simulink model "cm_commphasenoise"  (Simulink 10.1)
settings: Solver=FixedStepDiscrete  StartTime=0.0  StopTime=inf  RelTol=1e-3  EnableMultiTasking=on
PreLoadFcn:
  | Nbps = 8; % for 256 QAM
  | EbN0 = 35;
  | phaseNoise = -76;
  | freqOffset = 1000;
  | tgtMaxErr = 100;
libraries: commdigbbndam3 x2, commchan3 x1, commrandsrc3 x1, commsink2 x1, impairlib x1
Description:
  | Phase Noise Effects in 256-QAM
  | 
  | This model shows the effect of a receiver's phase noise on 256-ary quadrature amplitude modulation (QAM).
CloseFcn:
  | clear phnoiseSigsOut
  | 
  | % Close BER figure, if it exists
  | if exist('hPhaseNoise256QAM')  % figure has been created
  |     if ishandle(hPhaseNoise256QAM)  % figure still exists
  |         close(hPhaseNoise256QAM)
  |     end
  |     clear hPhaseNoise256QAM
  | end
settings Model: Creator=The MathWorks, Inc.  LastModifiedBy=iba  ExtModeAutoUpdateStatusClock=off
settings SolverCC: InsertRTBMode=Auto
settings DataIOCC: LimitDataPoints=on  SaveOutput=off  SaveTime=off  SignalLoggingName=phnoiseSigsOut
settings OptimizationCC: BlockReduction=off  BooleanDataType=off  ExpressionDepthLimit=2147483647  InitFltsAndDblsToZero=on  EfficientMapNaN2IntZero=off  BufferReusableBoundary=off
settings DebuggingCC: SaveWithParameterizedLinksMsg=none  CheckExecutionContextPreStartOutputMsg=on  CheckExecutionContextRuntimeOutputMsg=on  SignalResolutionControl=TryResolveAllWithWarning  InheritedTsInSrcMsg=none  MultiTaskDSMMsg=warning  MultiTaskCondExecSysMsg=none  SigSpecEnsureSampleTimeMsg=none  ParameterPrecisionLossMsg=none  FcnCallInpInsideContextMsg=warning  BusObjectLabelMismatch=none  StateNameClashWarn=warning
settings HardwareCC: TargetUnknown=on
settings ModelReferenceCC: UpdateModelReferenceTargets=IfOutOfDate
settings GRTTargetCC: TargetFcnLib=ansi_tfl_tmw.mat
settings ConfigComp: CovSFcnEnable=off

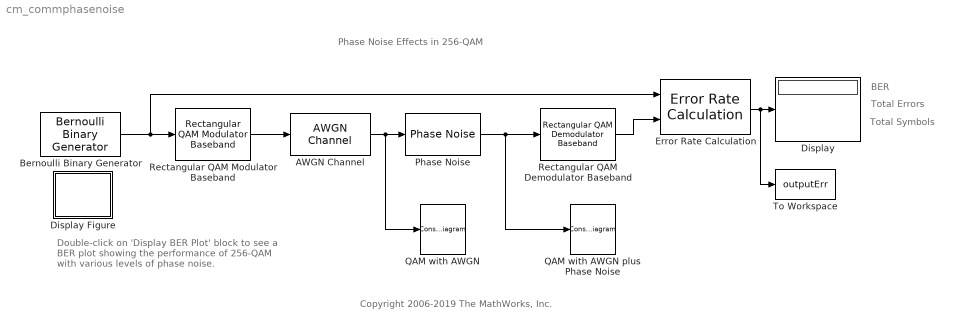
== system cm_commphasenoise ==
  note: Phase Noise Effects in 256-QAM
  note: Double-click on 'Display BER Plot' block
      | to see a BER plot showing the performance
      | of 256-QAM with various levels of phase noise.
  note: BER
  note: Total Errors
  note: Total Symbols
  note: Copyright 2006-2019 The MathWorks, Inc.
  AWGN Channel : commchan3/AWGN Channel  InputProcessing=Columns as channels (frame based)  seed=54321  noiseMode="Signal to noise ratio  (Eb/No)"  EbNodB=EbN0  EsNodB=40  SNRdB=10  bitsPerSym=Nbps  Ps=1  Tsym=1e-4*Nbps  variance=1
  Bernoulli Binary Generator : commrandsrc3/Bernoulli Binary Generator  ProbabilityOfZero=0.5  SeedSource=Auto  Seed=0  SampleTime=1e-4  SamplesPerFrame=Nbps*500  OutputDataType=boolean  SimulateUsing=Interpreted execution
  Display : Display
  Display Figure : Subsystem  mask(Display Figure){}
      settings: OpenFcn=commphasenoise_display;
      mask Display: disp('Display\nBER Plot');
  Error Rate Calculation : commsink2/Error Rate Calculation  N=0  st_delay=0  cp_mode=Entire frame  subframe=[]  PMode=Port  WsName=ErrorVec  RsMode2=off  stop=on  numErr=tgtMaxErr  maxBits=1e8
  Phase Noise : impairlib/Phase Noise  Level=phaseNoise  FrequencyOffset=freqOffset  SampleRate=10e3*Nbps  RandomStream=mt19937ar with seed  Seed=2137  SimulateUsing=Interpreted execution
      settings: SourceProductBaseCode=CM,AM,SX
  QAM with AWGN : ConstellationDiagram  Tag=ScatterPlot
  QAM with AWGN plus Phase Noise : ConstellationDiagram  Tag=ScatterPlot
  Rectangular QAM Demodulator Baseband : commdigbbndam3/Rectangular QAM Demodulator Baseband  M=2^Nbps  OutType=Bit  DecType=Hard decision  VarSource=Dialog  Variance=1  Dec=Binary  Mapping=[0:15]  PowType=Average Power  MinDist=2  AvgPow=1  PeakPow=1  Ph=0  outDtype1=boolean  outDtype2=uint8  derotateFactorWordLen=16  derotateFactorDataTypeStr=Inherit: Same word length as input  derotateFactorLastDataTypeStr=Inherit: Same word length as input  denormFactorWordLen=16  denormFactorDataTypeStr=Inherit: Same word length as input  denormFactorLastDataTypeStr=Inherit: Same word length as input  prodOutWordLen=32  prodOutOverflowMode=Wrap  prodOutRoundingMode=Floor  prodOutOvFlMode=off  prodOutOvFlModeLastStrValue=off  sumWordLen=32
  Rectangular QAM Modulator Baseband : commdigbbndam3/Rectangular QAM Modulator Baseband  M=2^Nbps  InType=Bit  Enc=Binary  Mapping=[0:15]  PowType=Average Power  MinDist=2  AvgPow=1  PeakPow=1  Ph=0  outDtype=single  outWordLen=16  outUDDataType=sfix(16)  outFracLenMode=Best precision  outFracLen=15  outDataTypeStr=single  outLastDataTypeStr=single
  To Workspace : ToWorkspace  VariableName=outputErr  SampleTime=-1
      settings: MaxDataPoints=1  Save2DSignal=2-D array (concatenate along first dimension)
  wires:
  AWGN Channel/1 -> QAM with AWGN/1, Phase Noise/1
  Rectangular QAM Modulator Baseband/1 -> AWGN Channel/1
  Phase Noise/1 -> Rectangular QAM Demodulator Baseband/1, QAM with AWGN plus Phase Noise/1
  Rectangular QAM Demodulator Baseband/1 -> Error Rate Calculation/2
  Error Rate Calculation/1 -> To Workspace/1, Display/1
  Bernoulli Binary Generator/1 -> Error Rate Calculation/1, Rectangular QAM Modulator Baseband/1

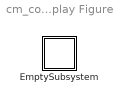
== system cm_commphasenoise/Display Figure ==
  EmptySubsystem : Subsystem

== system cm_commphasenoise/Display Figure/EmptySubsystem ==
